simulink model "sldemo_ifsub"  (Simulink 7.6)
settings: Solver=VariableStepDiscrete  StartTime=0.0  StopTime=10.0  RelTol=1e-3
StartFcn:
  | set_param('sldemo_ifsub/Scope','Open','on');
Description:
  | If-Then-Else Blocks
  | 
  | This demonstration shows what happens when a sine wave is fed into an
  | If block.  After running the simulation, the scope shows three plots.  This
  | demonstration is designed to compare the If block with enabled subsystems.
  | 
  | The first of these plots shows the original sine wave and the absolute
  | value of the original sine wave offset by two.  The absolute value of the sine
  | wave is only shown when the subsystem is executed.  This occurs between
  | 0 and 2.5 seconds and 5 and 7.5 seconds.  When the subsystem is not
  | executed then the output of the subsystem is reset to 0.  The value of 0 is
  | determined by the initial condition of the outport. You can see when
  | the subsystem is executed by looking at the second plot.  A value of 1
  | indicates that it is executed.
  | 
  | The second plot shows the original value of the input signal.  If the signal
  | is towards the top of the plot then the if subsystem related to the first plot
  | is executed.  If the signal is towards the bottom of the plot then the else
  | subsystem related to the third plot is executed.
  | 
  | The third plot shows the original sine wave and the saturation limited sine
  | wave offset by two.  The saturated value of the sine wave is only shown when
  | the subsystem is executed.  This occurs between 2.5 and 5 seconds and 7.5
  | and 10 seconds.
settings Model: Creator=The MathWorks Inc.  CovMetricSettings=d  ExtModeTrigMode=oneshot  ExtModeArmWhenConnect=off  ExtModeAutoUpdateStatusClock=off
settings DataIOCC: LimitDataPoints=off  SaveOutput=off  SaveTime=off
settings OptimizationCC: BlockReduction=off  BooleanDataType=off  InlineInvariantSignals=on  InitFltsAndDblsToZero=on  BufferReusableBoundary=off
settings DebuggingCC: SaveWithParameterizedLinksMsg=none  SignalResolutionControl=TryResolveAllWithWarning  SolverPrmCheckMsg=none  MultiTaskDSMMsg=warning  MultiTaskCondExecSysMsg=none  SigSpecEnsureSampleTimeMsg=none  IntegerOverflowMsg=none  BusObjectLabelMismatch=none
settings HardwareCC: TargetUnknown=on
settings RTWCC: IncludeERTFirstTime=on
settings GRTTargetCC: TargetFcnLib=ansi_tfl_tmw.mat

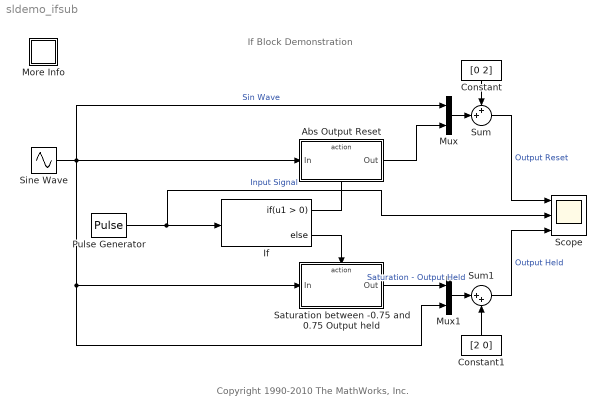
== system sldemo_ifsub ==
  note: If Block Demonstration
  note: Copyright 1990-2010 The MathWorks, Inc.
  Abs Output Reset : Subsystem  TreatAsAtomicUnit=on
  Constant : Constant  Value=[0 2]
  Constant1 : Constant  Value=[2 0]
  If : If
  More Info : Subsystem
      settings: OpenFcn=showdemo(bdroot(gcb))
      mask Display: disp('?')
  Mux : Mux  Inputs=2
  Mux1 : Mux  Inputs=2
  Pulse Generator : DiscretePulseGenerator  PulseType=Time based  Period=5  PulseWidth=50
      settings: AttributesFormatString=Period: %<period>\nDuty cycle: %<pulsewidth>%
  Saturation between -0.75 and 0.75 Output held : Subsystem  TreatAsAtomicUnit=on
  Scope : Scope  NumInputPorts=3
      settings: StartFcn=open_system(gcbh)  TickLabels=on  TimeRange=10  YMin=-1.6~-0.1~-1.5  YMax=3.6~1.1~3.5  DataFormat=Structure
  Sine Wave : Sin  SampleTime=0
  Sum : Sum  Inputs=++|  SaturateOnIntegerOverflow=on  InputSameDT=on  OutDataTypeStr=Inherit: Same as first input
  Sum1 : Sum  Inputs=|++  SaturateOnIntegerOverflow=on  InputSameDT=on  OutDataTypeStr=Inherit: Same as first input
  wires:
  Sine Wave/1 -> Abs Output Reset/1(In), Mux/1, Saturation between -0.75 and 0.75 Output held/1(In), Mux1/2  "Sin Wave"
  Saturation between -0.75 and 0.75 Output held/1(Out) -> Mux1/1  "Saturation - Output Held"
  Constant/1 -> Sum/1
  Mux/1 -> Sum/2
  Abs Output Reset/1(Out) -> Mux/2
  Sum/1 -> Scope/1  "Output Reset"
  Mux1/1 -> Sum1/1
  Constant1/1 -> Sum1/2
  Sum1/1 -> Scope/3  "Output Held"
  Pulse Generator/1 -> If/1, Scope/2  "Input Signal"
  If/2 -> Saturation between -0.75 and 0.75 Output held/Action
  If/1 -> Abs Output Reset/Action

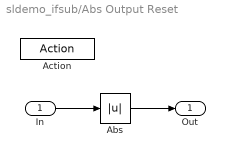
== system sldemo_ifsub/Abs Output Reset ==
  In : Inport
  Action : ActionPort  InitializeStates=reset  ActionType=then
  Abs : Abs  SaturateOnIntegerOverflow=on
  Out : Outport  OutputWhenDisabled=reset  InitialOutput=0
  wires:
  In/1 -> Abs/1
  Abs/1 -> Out/1

== system sldemo_ifsub/More Info ==

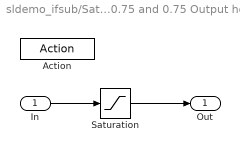
== system sldemo_ifsub/Saturation between -0.75 and 0.75 Output held ==
  In : Inport
  Action : ActionPort  ActionType=else
  Saturation : Saturate  UpperLimit=0.75  LowerLimit=-0.75
  Out : Outport
  wires:
  Saturation/1 -> Out/1
  In/1 -> Saturation/1
